simulink model "keypad_DONE"  (R2019b)
settings: Solver=ode1  StartTime=0.0  StopTime=inf  FixedStep=0.01  RelTol=1e-3  EnableMultiTasking=on
libraries: arduinolib x3
settings Model: ExtModeTrigDuration=2  Creator=estra  LastModifiedBy=fabia
settings DataIOCC: ReturnWorkspaceOutputs=off
settings OptimizationCC: MaxStackSize=64  EfficientTunableParamExpr=on
settings DebuggingCC: ParameterTunabilityLossMsg=error  ArithmeticOperatorsInVariantConditions=warning
settings HardwareCC: ProdBitPerInt=16  ProdBitPerPointer=16  ProdBitPerSizeT=16  ProdBitPerPtrDiffT=16  ProdLargestAtomicFloat=None  ProdWordSize=8  ProdHWDeviceType=Atmel->AVR
settings SFSimCC: SimUseLocalCustomCode=off  MATLABDynamicMemAlloc=off  CustomCodeUndefinedFunction=UseInterfaceOnly
settings RTWCC: SystemTargetFile=ert.tlc  HardwareBoard=Arduino Uno  TLCOptions=-aInlineSetEventsForThisBaseRateFcn=TLC_FALSE -aSuppressMultiTaskScheduler=TLC_FALSE -aRateBasedStepFcn=1  TemplateMakefile=ert_default_tmf  GenerateReport=on  RTWUseLocalCustomCode=off  Toolchain=Arduino AVR  BuildConfiguration=Faster Runs  IncludeHyperlinkInReport=on  LaunchReport=on  GenerateTraceInfo=on  GenerateTraceReport=on  GenerateTraceReportSl=on  GenerateTraceReportSf=on  GenerateTraceReportEml=on
settings CodeAppCC: ForceParamTrailComments=on  IgnoreCustomStorageClasses=off  OperatorAnnotations=on  SimulinkDataObjDesc=on  SFDataObjDesc=on  MATLABFcnDesc=on  InsertBlockDesc=on  StateflowObjectComments=on  MATLABSourceComments=on
settings ERTTargetCC: MultiwordLength=2048  SupportContinuousTime=on  SupportVariableSizeSignals=on

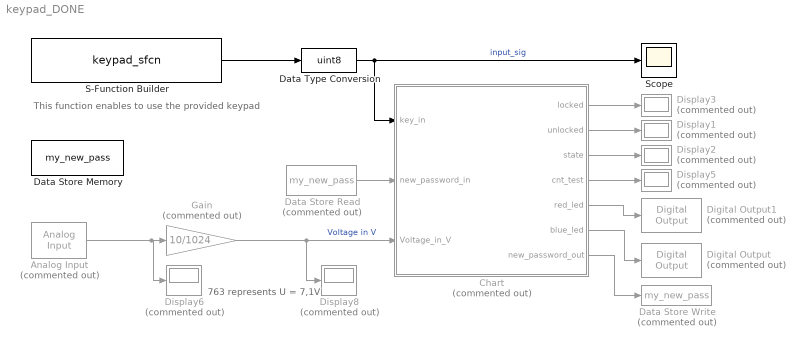
== system keypad_DONE ==
  note: 763 represents U = 7,1V
  note: This function enables to use the provided keypad
  Analog Input : arduinolib/Analog Input  Commented=on  pinNumber=0  ReadResultsOnly=off  ConversionTriggerSource=Software  ExternalTriggerType=uint32(0)  OutputDataType=uint16  EnableConversionCompleteNotify=off  EnableOuputStatus=off  SampleTime=-1  blockPlatform=arduino
  Chart : Stateflow chart  Commented=on  BlockKeywords=__PRM__SERIALIZED__DATA__:Stateflow Chart,Stateflow Diagram  TreatAsAtomicUnit=on
  Data Store Read : DataStoreRead  Commented=on  DataStoreName=my_new_pass
  Data Store Write : DataStoreWrite  Commented=on  DataStoreName=my_new_pass
  Data Store Memory : DataStoreMemory  DataStoreName=my_new_pass  ReadBeforeWriteMsg=warning  WriteAfterWriteMsg=warning  WriteAfterReadMsg=warning  InitialValue=[1 1 1 1 1 1]  ShowAdditionalParam=off  OutDataTypeStr=int8
  Data Type Conversion : DataTypeConversion  OutDataTypeStr=uint8
  Digital Output : arduinolib/Digital Output  Commented=on  pinNumber=13  blockPlatform=arduino
  Digital Output1 : arduinolib/Digital Output  Commented=on  pinNumber=12  blockPlatform=arduino
  Display{1..3,5..6,8} (6 alike) : Display  Commented=on
  Gain : Gain  Commented=on  Gain=10/1024
  S-Function Builder : S-Function  InitFcn=try, set_param(gcb,'FunctionName','keypad_sfcn'), end  FunctionName=keypad_sfcn  SFunctionModules=keypad_sfcn_wrapper  SFunctionDeploymentMode=off  EnableBusSupport=off  mask(S-Function Builder){}
      mask help: Simulink:masks:SFunctionBuilder_MD
      mask init:
      | val = [[.9  0.75 0.75 1 1 .9 .9 1]',[1 1 0.75 0.75 .9 .9 1 .9]'];try , sys = get_param(gcb,'SfunBuilderFcnName');if isempty(sys), sys = get_param(gcb,'FunctionName'); end,catch, sys = get_param(gcb,'FunctionName'); end
      settings: CopyFcn=set_param(gcbh,'LinkStatus','none')  PreSaveFcn=try, set_param(gcb,'FunctionName','keypad_sfcn'), end  OpenFcn=sfunctionwizard(gcbh)
      mask Display: plot(val(:,1),val(:,2)),disp(sys), port_label('output',1,'y0')
  Scope : Scope
  wires:
  Data Type Conversion/1 -> Chart/1(key_in), Scope/1  "input_sig"
  Chart/3(state) -> Display2/1
  Chart/1(locked) -> Display3/1
  Chart/4(cnt_test) -> Display5/1
  Chart/6(blue_led) -> Digital Output/1
  Chart/2(unlocked) -> Display1/1
  Analog Input/1 -> Display6/1, Gain/1
  Gain/1 -> Display8/1, Chart/3(Voltage_in_V)  "Voltage in V"
  Chart/5(red_led) -> Digital Output1/1
  S-Function Builder/1 -> Data Type Conversion/1
  Data Store Read/1 -> Chart/2(new_password_in)
  Chart/7(new_password_out) -> Data Store Write/1

== stateflow chart keypad_DONE/Chart ==
  settings: executeAtInitialization=1
  state DEFAULT_VAL
    entry:
    new_password_out = [1 1 1 1 1 1];
    state = 15;
  state INIT
    correct_password = new_password_in;
    password_in = [0 0 0 0 0 0];
    cnt = 0;
    index = 1;
    unlocked = 0;
    key_dec = 0;
    exit_key = 0;
    state = 0;
    cnt_test = 1;
    zero = 0;
    red_led = false;
    blue_led = false;
    flag_new_pass = false;
  state SET_NEW_PASS2
    entry:
    exit_key = 0;
    during:
    state = 17;
    cnt_test = index;
    exit_key = int8(key_in)- int8(48);
  state LOW_BAT
    entry:
    state = 18;
    red_led = true;
    blue_led = true;
  state SET_NEW_PASS1
    entry:
    flag_new_pass = true;
    new_password_out(index) = int8(key_in)- int8(48);
    state = 16;
    cnt_test = index;
    exit:
    index = index+1;
  state IDLE
    % just wait
    entry:
    state = 1;
    red_led = true;
  state CONVERT
    %key_dec = ascii_to_dec(key_in);
    key_dec = int8(key_in) - int8(48);
    state = 2;
  state CHECK_CONFIRMATION % # = -13
    entry:
    confirm_key = 0;
    during:
    confirm_key = key_dec;
    state = 6;
  state INPUT_HANDLING
    entry:
    password_in(index) = key_dec;
    index = index+1;
    cnt_test = index;
    exit:
    state = 3;
  state CHECK_SEQ
    during:
    state = 4;
  state WRONG_SEQ
    entry:
    red_led = false;
    cnt = cnt + 1;
    unlocked = 0;
    locked = 1;
    exit:
    cnt_blink = 0;
    index = 1;
    state = 7;
  state RIGHT_SEQ
    entry:
    exit_key = 0;
    cnt_test = 33;
    flag_new_pass = true;
    during:
    blue_led = true;
    red_led = false;
    exit_key = int8(key_in)- int8(48);
    unlocked = 1;
    locked = 0;
    index = 1;
    state = 9;
    exit:
    blue_led = false;
  state BLINK_RED1
    entry:
    red_led =~ red_led;
  state BLINK_RED2
    entry:
    red_led =~ red_led;
    exit:
    red_led = true;
  state BLOCKING
    entry:
    cnt = 0;
    during:
    exit_key = int8(key_in) - int8(48);
    state = 8;
  state BLOCKING_BLINK
    entry:
    cnt_blink = cnt_blink + 1;
    red_led = ~red_led;
    blue_led =~blue_led;
    during:
    exit_key = int8(key_in) - int8(48)
    state = 11;
  (default) -> DEFAULT_VAL
  DEFAULT_VAL -> INIT
  RIGHT_SEQ -> SET_NEW_PASS2 [order 2] : [exit_key == -6]
  IDLE -> LOW_BAT [order 2] : [Voltage_in_V < 5]
  SET_NEW_PASS2 -> INIT [order 1] : [hasChangedTo(key_in, uint8(35))]
  LOW_BAT -> IDLE : after(1, sec)
  BLOCKING_BLINK -> INIT [order 2] : [exit_key == -6]
  SET_NEW_PASS2 -> SET_NEW_PASS1 [order 2] : [(hasChangedFrom(key_in, zero))]
  SET_NEW_PASS1 -> SET_NEW_PASS2 : after(0.1, sec)
  BLOCKING -> INIT [order 1] : [(exit_key == -6) || (after(20,sec)) || cnt_blink == 20]
  RIGHT_SEQ -> INIT [order 1] : [ (after(20, sec)) || (exit_key == 17) ]
  INIT -> IDLE
  INPUT_HANDLING -> IDLE
  BLINK_RED2 -> IDLE [order 1] : after(0.5, sec)
  IDLE -> CONVERT [order 1] : [hasChangedFrom(key_in, zero)]
  CONVERT -> INPUT_HANDLING [order 1] : [(key_dec ~= -13) && (flag_new_pass == false) ]
  CONVERT -> CHECK_CONFIRMATION % # = -13 [order 2] : [key_dec == -13]
  CHECK_CONFIRMATION % # = -13 -> CHECK_SEQ : [confirm_key == -13]
  CHECK_SEQ -> WRONG_SEQ [order 2] : [compare(password_in, correct_password) == 0]
  CHECK_SEQ -> RIGHT_SEQ [order 1] : [compare(password_in, correct_password) == 1]
  WRONG_SEQ -> BLINK_RED1 : after(0.5, sec)
  BLINK_RED1 -> BLINK_RED2 : after(0.5, sec)
  BLINK_RED2 -> BLOCKING [order 2] : [cnt == 3]
  BLOCKING_BLINK -> BLOCKING [order 1] : after(0.5,sec)
  BLOCKING -> BLOCKING_BLINK [order 2] : after(0.5, sec)
  data: key_in input uint8; locked output uint8; unlocked output uint8; cnt local uint8; index local uint8; correct_password local; password_in local; state output uint8; key_dec local int8; confirm_key local int8; exit_key local int8; cnt_test output uint8; zero local uint8; red_led output boolean; blue_led output boolean; cnt_blink local; my_new_pass data_store_memory; new_password_in input int8 size=[1 6]; new_password_out output int8 size=[1 6]; Voltage_in_V input
